simulink model "Bicycle_model_unconstrained"  (R2020b)
settings: Solver=ode15s  StartTime=0.0  StopTime=10.0  RelTol=1e-3
libraries: simulink_extras x4
settings Model: Creator=yafta  LastModifiedBy=Matthew

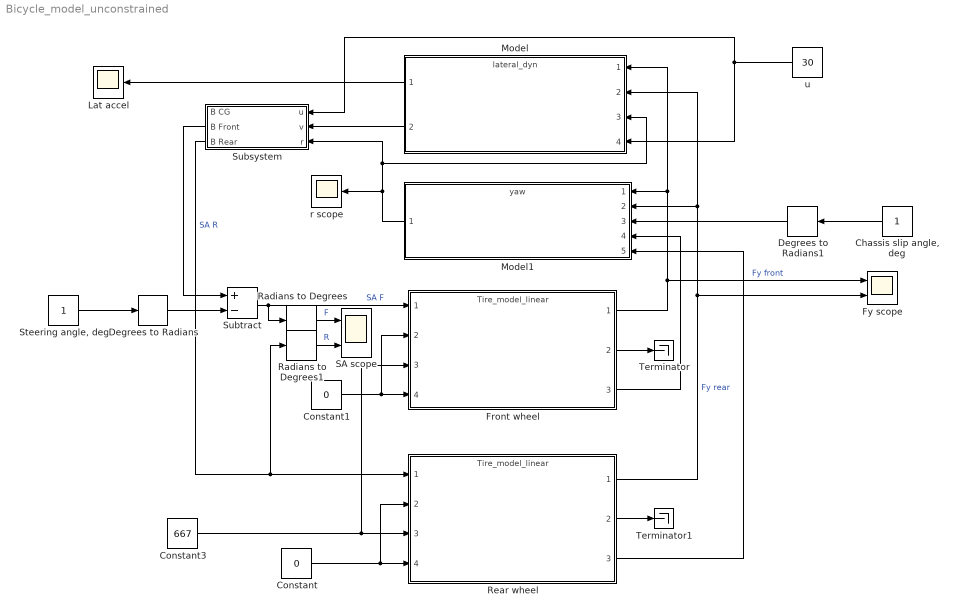
== system Bicycle_model_unconstrained ==
  "Chassis slip angle, deg" : Constant
  Constant : Constant  Value=0
  Constant1 : Constant  Value=0
  Constant3 : Constant  Value=667
  Degrees to Radians : simulink_extras/Transformations/Degrees to Radians
  Degrees to Radians1 : simulink_extras/Transformations/Degrees to Radians
  Front wheel : ModelReference  ModelNameDialog=Tire_model_linear  SimulationMode=Normal  ModelReferenceVersion=2.4
  Fy scope : Scope  NumInputPorts=2
  Lat accel : Scope
  Model : ModelReference  ModelNameDialog=lateral_dyn.slx  SimulationMode=Normal  ModelReferenceVersion=2.1
  Model1 : ModelReference  ModelNameDialog=yaw.slx  SimulationMode=Normal  ModelReferenceVersion=2.4
  Radians to Degrees : simulink_extras/Transformations/Radians to Degrees
  Radians to Degrees1 : simulink_extras/Transformations/Radians to Degrees
  Rear wheel : ModelReference  ModelNameDialog=Tire_model_linear  SimulationMode=Normal  ModelReferenceVersion=2.4
  SA scope : Scope  NumInputPorts=2
  "Steering angle, deg" : Constant
  Subsystem : Subsystem
  Subtract : Sum  Inputs=+-
  Terminator : Terminator
  Terminator1 : Terminator
  r scope : Scope
  u : Constant  Value=30
  wires:
  Constant/1 -> Rear wheel/4, Rear wheel/2
  Constant1/1 -> Front wheel/2, Front wheel/4
  Front wheel/2 -> Terminator/1
  Rear wheel/2 -> Terminator1/1
  Rear wheel/1 -> Fy scope/2, Model1/2, Model/2  "Fy rear"
  Model1/1 -> Subsystem/3(r), Model/3, r scope/1
  Front wheel/1 -> Model/1, Model1/1, Fy scope/1  "Fy front"
  Model/2 -> Subsystem/2(v)
  u/1 -> Model/4, Subsystem/1(u)
  Subsystem/2(B Front) -> Subtract/1
  "Steering angle, deg"/1 -> Degrees to Radians/1
  Subtract/1 -> Radians to Degrees/1, Front wheel/1  "SA F"
  Subsystem/3(B Rear) -> Radians to Degrees1/1, Rear wheel/1  "SA R"
  "Chassis slip angle, deg"/1 -> Degrees to Radians1/1
  Model/1 -> Lat accel/1
  Constant3/1 -> Rear wheel/3, Front wheel/3
  Front wheel/3 -> Model1/4
  Rear wheel/3 -> Model1/5
  Degrees to Radians/1 -> Subtract/2
  Degrees to Radians1/1 -> Model1/3
  Radians to Degrees/1 -> SA scope/1  "F"
  Radians to Degrees1/1 -> SA scope/2  "R"

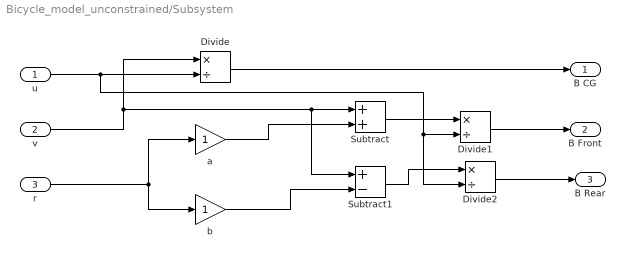
== system Bicycle_model_unconstrained/Subsystem ==
  u : Inport
  v : Inport  Port=2
  r : Inport  Port=3
  Divide : Product  Inputs=*/
  Divide1 : Product  Inputs=*/
  Divide2 : Product  Inputs=*/
  Subtract : Sum
  Subtract1 : Sum  Inputs=+-
  a : Gain
  b : Gain
  B CG : Outport
  B Front : Outport  Port=2
  B Rear : Outport  Port=3
  wires:
  v/1 -> Subtract1/1, Subtract/1, Divide/1
  u/1 -> Divide2/2, Divide1/2, Divide/2
  Divide/1 -> B CG/1
  r/1 -> a/1, b/1
  a/1 -> Subtract/2
  b/1 -> Subtract1/2
  Subtract/1 -> Divide1/1
  Subtract1/1 -> Divide2/1
  Divide1/1 -> B Front/1
  Divide2/1 -> B Rear/1
